simulink model "automata_learning"  (R2022a)
(part 8 of 10)

(exp(0.7734684944152832 * x2 - 0.6509665846824646 * x1 + 0.04056214913725853) - 1.0) / (exp(0.7734684944152832 * x2 - 0.6509665846824646 * x1 + 0.04056214913725853) + 1.0) + 0.0358128547668457 * (exp(0.018543146550655365 * x2 - 0.7226533889770508 * x1 + 0.3809460401535034) - 1.0) / (exp(0.018543146550655365 * x2 - 0.7226533889770508 * x1 + 0.3809460401535034) + 1.0) + 0.16037598252296448 * (exp(0.03828786686062813 * x1 + 0.43738114833831787 * x2 - 0.15343865752220154) - 1.0) / (exp(0.03828786686062813 * x1 + 0.43738114833831787 * x2 - 0.15343865752220154) + 1.0) + 0.879189133644104 * (exp(0.3266531825065613 * x1 + 0.7609410881996155 * x2 + 0.40537890791893005) - 1.0) / (exp(0.3266531825065613 * x1 + 0.7609410881996155 * x2 + 0.40537890791893005) + 1.0) + 0.47213396430015564 * (exp(0.20762847363948822 * x1 + 0.2858797609806061 * x2 - 0.43727564811706543) - 1.0) / (exp(0.20762847363948822 * x1 + 0.2858797609806061 * x2 - 0.43727564811706543) + 1.0) - 0.3890422284603119 * (exp(0.005666637327522039 * x1 + 0.6119794845581055 * x2 - 0.9893868565559387) - 1.0) / (exp(0.005666637327522039 * x1 + 0.6119794845581055 * x2 - 0.9893868565559387) + 1.0) + 0.4245724678039551 * (exp(0.39608341455459595 * x1 + 0.04428500309586525 * x2 + 0.2183447629213333) - 1.0) / (exp(0.39608341455459595 * x1 + 0.04428500309586525 * x2 + 0.2183447629213333) + 1.0) - 0.5148495435714722 * (exp(0.5634458065032959 * x1 - 0.8322378396987915 * x2 + 0.24965126812458038) - 1.0) / (exp(0.5634458065032959 * x1 - 0.8322378396987915 * x2 + 0.24965126812458038) + 1.0) - 0.5015235543251038 * (exp(0.3741709291934967 * x1 - 0.829635500907898 * x2 + 0.40845659375190735) - 1.0) / (exp(0.3741709291934967 * x1 - 0.829635500907898 * x2 + 0.40845659375190735) + 1.0) - 0.5266704559326172 * (exp(0.11800816655158997 * x2 - 0.6871803402900696 * x1 + 0.20091386139392853) - 1.0) / (exp(0.11800816655158997 * x2 - 0.6871803402900696 * x1 + 0.20091386139392853) + 1.0) - 0.6838598847389221 * (exp(0.19844788312911987 * x1 + 0.4046936631202698 * x2 - 0.9344500303268433) - 1.0) / (exp(0.19844788312911987 * x1 + 0.4046936631202698 * x2 - 0.9344500303268433) + 1.0) + 0.32724878191947937) + 1.0) - 0.29631882905960083 * (exp(0.33656391501426697 * (exp(0.5020318031311035 * x2 - 0.13788816332817078 * x1 + 0.02421402372419834) - 1.0) / (exp(0.5020318031311035 * x2 - 0.13788816332817078 * x1 + 0.02421402372419834) + 1.0) + 0.2108035683631897 * (exp(0.6166407465934753 * x1 + 1.262364149093628 * x2 + 0.2914634048938751) - 1.0) / (exp(0.6166407465934753 * x1 + 1.262364149093628 * x2 + 0.2914634048938751) + 1.0) + 0.5500431656837463 * (exp(0.03550431877374649 * x1 + 0.5916184186935425 * x2 - 0.08759552985429764) - 1.0) / (exp(0.03550431877374649 * x1 + 0.5916184186935425 * x2 - 0.08759552985429764) + 1.0) + 0.29068365693092346 * (exp(0.1657479703426361 * x1 - 0.679574728012085 * x2 + 0.5307417511940002) - 1.0) / (exp(0.1657479703426361 * x1 - 0.679574728012085 * x2 + 0.5307417511940002) + 1.0) + 0.6584247946739197 * (exp(0.14132575690746307 * x1 - 0.739913821220398 * x2 + 1.2046058177947998) - 1.0) / (exp(0.14132575690746307 * x1 - 0.739913821220398 * x2 + 1.2046058177947998) + 1.0) + 0.5027154088020325 * (exp(0.6150497794151306 * x1 - 0.6773995757102966 * x2 + 0.330721378326416) - 1.0) / (exp(0.6150497794151306 * x1 - 0.6773995757102966 * x2 + 0.330721378326416) + 1.0) - 0.6585365533828735 * (exp(0.3733357787132263 * x1 - 0.6249079704284668 * x2 + 0.3175375759601593) - 1.0) / (exp(0.3733357787132263 * x1 - 0.6249079704284668 * x2 + 0.3175375759601593) + 1.0) + 0.7110286951065063 * (exp(1.5124197006225586 * x1 + 1.2726414203643799 * x2 + 1.264981746673584) - 1.0) / (exp(1.5124197006225586 * x1 + 1.2726414203643799 * x2 + 1.264981746673584) + 1.0) + 0.14636917412281036 * (exp(0.6106719970703125 * x2 - 0.2651570439338684 * x1 + 0.22832649946212769) - 1.0) / (exp(0.6106719970703125 * x2 - 0.2651570439338684 * x1 + 0.22832649946212769) + 1.0) + 0.31852221488952637 * (exp(0.7734684944152832 * x2 - 0.6509665846824646 * x1 + 0.04056214913725853) - 1.0) / (exp(0.7734684944152832 * x2 - 0.6509665846824646 * x1 + 0.04056214913725853) + 1.0) + 0.049165740609169006 * (exp(0.018543146550655365 * x2 - 0.7226533889770508 * x1 + 0.3809460401535034) - 1.0) / (exp(0.018543146550655365 * x2 - 0.7226533889770508 * x1 + 0.3809460401535034) + 1.0) - 0.2836047410964966 * (exp(0.03828786686062813 * x1 + 0.43738114833831787 * x2 - 0.15343865752220154) - 1.0) / (exp(0.03828786686062813 * x1 + 0.43738114833831787 * x2 - 0.15343865752220154) + 1.0) - 0.5415816307067871 * (exp(0.3266531825065613 * x1 + 0.7609410881996155 * x2 + 0.40537890791893005) - 1.0) / (exp(0.3266531825065613 * x1 + 0.7609410881996155 * x2 + 0.40537890791893005) + 1.0) - 0.4399423599243164 * (exp(0.20762847363948822 * x1 + 0.2858797609806061 * x2 - 0.43727564811706543) - 1.0) / (exp(0.20762847363948822 * x1 + 0.2858797609806061 * x2 - 0.43727564811706543) + 1.0) - 0.0010141741950064898 * (exp(0.005666637327522039 * x1 + 0.6119794845581055 * x2 - 0.9893868565559387) - 1.0) / (exp(0.005666637327522039 * x1 + 0.6119794845581055 * x2 - 0.9893868565559387) + 1.0) + 0.5742956399917603 * (exp(0.39608341455459595 * x1 + 0.04428500309586525 * x2 + 0.2183447629213333) - 1.0) / (exp(0.39608341455459595 * x1 + 0.04428500309586525 * x2 + 0.2183447629213333) + 1.0) - 0.03165071830153465 * (exp(0.5634458065032959 * x1 - 0.8322378396987915 * x2 + 0.24965126812458038) - 1.0) / (exp(0.5634458065032959 * x1 - 0.8322378396987915 * x2 + 0.24965126812458038) + 1.0) - 0.6148557066917419 * (exp(0.3741709291934967 * x1 - 0.829635500907898 * x2 + 0.40845659375190735) - 1.0) / (exp(0.3741709291934967 * x1 - 0.829635500907898 * x2 + 0.40845659375190735) + 1.0) - 0.4349830448627472 * (exp(0.11800816655158997 * x2 - 0.6871803402900696 * x1 + 0.20091386139392853) - 1.0) / (exp(0.11800816655158997 * x2 - 0.6871803402900696 * x1 + 0.20091386139392853) + 1.0) + 0.4710049331188202 * (exp(0.19844788312911987 * x1 + 0.4046936631202698 * x2 - 0.9344500303268433) - 1.0) / (exp(0.19844788312911987 * x1 + 0.4046936631202698 * x2 - 0.9344500303268433) + 1.0) + 0.1878088265657425) - 1.0) / (exp(0.33656391501426697 * (exp(0.5020318031311035 * x2 - 0.13788816332817078 * x1 + 0.02421402372419834) - 1.0) / (exp(0.5020318031311035 * x2 - 0.13788816332817078 * x1 + 0.02421402372419834) + 1.0) + 0.2108035683631897 * (exp(0.6166407465934753 * x1 + 1.262364149093628 * x2 + 0.2914634048938751) - 1.0) / (exp(0.6166407465934753 * x1 + 1.262364149093628 * x2 + 0.2914634048938751) + 1.0) + 0.5500431656837463 * (exp(0.03550431877374649 * x1 + 0.5916184186935425 * x2 - 0.08759552985429764) - 1.0) / (exp(0.03550431877374649 * x1 + 0.5916184186935425 * x2 - 0.08759552985429764) + 1.0) + 0.29068365693092346 * (exp(0.1657479703426361 * x1 - 0.679574728012085 * x2 + 0.5307417511940002) - 1.0) / (exp(0.1657479703426361 * x1 - 0.679574728012085 * x2 + 0.5307417511940002) + 1.0) + 0.6584247946739197 * (exp(0.14132575690746307 * x1 - 0.739913821220398 * x2 + 1.2046058177947998) - 1.0) / (exp(0.14132575690746307 * x1 - 0.739913821220398 * x2 + 1.2046058177947998) + 1.0) + 0.5027154088020325 * (exp(0.6150497794151306 * x1 - 0.6773995757102966 * x2 + 0.330721378326416) - 1.0) / (exp(0.6150497794151306 * x1 - 0.6773995757102966 * x2 + 0.330721378326416) + 1.0) - 0.6585365533828735 * (exp(0.3733357787132263 * x1 - 0.6249079704284668 * x2 + 0.3175375759601593) - 1.0) / (exp(0.3733357787132263 * x1 - 0.6249079704284668 * x2 + 0.3175375759601593) + 1.0) + 0.7110286951065063 * (exp(1.5124197006225586 * x1 + 1.2726414203643799 * x2 + 1.264981746673584) - 1.0) / (exp(1.5124197006225586 * x1 + 1.2726414203643799 * x2 + 1.264981746673584) + 1.0) + 0.14636917412281036 * (exp(0.6106719970703125 * x2 - 0.2651570439338684 * x1 + 0.22832649946212769) - 1.0) / (exp(0.6106719970703125 * x2 - 0.2651570439338684 * x1 + 0.22832649946212769) + 1.0) + 0.31852221488952637 * (exp(0.7734684944152832 * x2 - 0.6509665846824646 * x1 + 0.04056214913725853) - 1.0) / (exp(0.7734684944152832 * x2 - 0.6509665846824646 * x1 + 0.04056214913725853) + 1.0) + 0.049165740609169006 * (exp(0.018543146550655365 * x2 - 0.7226533889770508 * x1 + 0.3809460401535034) - 1.0) / (exp(0.018543146550655365 * x2 - 0.7226533889770508 * x1 + 0.3809460401535034) + 1.0) - 0.2836047410964966 * (exp(0.03828786686062813 * x1 + 0.43738114833831787 * x2 - 0.15343865752220154) - 1.0) / (exp(0.03828786686062813 * x1 + 0.43738114833831787 * x2 - 0.15343865752220154) + 1.0) - 0.5415816307067871 * (exp(0.3266531825065613 * x1 + 0.7609410881996155 * x2 + 0.40537890791893005) - 1.0) / (exp(0.3266531825065613 * x1 + 0.7609410881996155 * x2 + 0.40537890791893005) + 1.0) - 0.4399423599243164 * (exp(0.20762847363948822 * x1 + 0.2858797609806061 * x2 - 0.43727564811706543) - 1.0) / (exp(0.20762847363948822 * x1 + 0.2858797609806061 * x2 - 0.43727564811706543) + 1.0) - 0.0010141741950064898 * (exp(0.005666637327522039 * x1 + 0.6119794845581055 * x2 - 0.9893868565559387) - 1.0) / (exp(0.005666637327522039 * x1 + 0.6119794845581055 * x2 - 0.9893868565559387) + 1.0) + 0.5742956399917603 * (exp(0.39608341455459595 * x1 + 0.04428500309586525 * x2 + 0.2183447629213333) - 1.0) / (exp(0.39608341455459595 * x1 + 0.04428500309586525 * x2 + 0.2183447629213333) + 1.0) - 0.03165071830153465 * (exp(0.5634458065032959 * x1 - 0.8322378396987915 * x2 + 0.24965126812458038) - 1.0) / (exp(0.5634458065032959 * x1 - 0.8322378396987915 * x2 + 0.24965126812458038) + 1.0) - 0.6148557066917419 * (exp(0.3741709291934967 * x1 - 0.829635500907898 * x2 + 0.40845659375190735) - 1.0) / (exp(0.3741709291934967 * x1 - 0.829635500907898 * x2 + 0.40845659375190735) + 1.0) - 0.4349830448627472 * (exp(0.11800816655158997 * x2 - 0.6871803402900696 * x1 + 0.20091386139392853) - 1.0) / (exp(0.11800816655158997 * x2 - 0.6871803402900696 * x1 + 0.20091386139392853) + 1.0) + 0.4710049331188202 * (exp(0.19844788312911987 * x1 + 0.4046936631202698 * x2 - 0.9344500303268433) - 1.0) / (exp(0.19844788312911987 * x1 + 0.4046936631202698 * x2 - 0.9344500303268433) + 1.0) + 0.1878088265657425) + 1.0) - 0.2150561660528183 * (exp(0.02026395872235298 * (exp(0.6166407465934753 * x1 + 1.262364149093628 * x2 + 0.2914634048938751) - 1.0) / (exp(0.6166407465934753 * x1 + 1.262364149093628 * x2 + 0.2914634048938751) + 1.0) - 0.03688286617398262 * (exp(0.5020318031311035 * x2 - 0.13788816332817078 * x1 + 0.02421402372419834) - 1.0) / (exp(0.5020318031311035 * x2 - 0.13788816332817078 * x1 + 0.02421402372419834) + 1.0) + 0.8227269649505615 * (exp(0.03550431877374649 * x1 + 0.5916184186935425 * x2 - 0.08759552985429764) - 1.0) / (exp(0.03550431877374649 * x1 + 0.5916184186935425 * x2 - 0.08759552985429764) + 1.0) + 0.10660602152347565 * (exp(0.1657479703426361 * x1 - 0.679574728012085 * x2 + 0.5307417511940002) - 1.0) / (exp(0.1657479703426361 * x1 - 0.679574728012085 * x2 + 0.5307417511940002) + 1.0) + 0.0043801916763186455 * (exp(0.14132575690746307 * x1 - 0.739913821220398 * x2 + 1.2046058177947998) - 1.0) / (exp(0.14132575690746307 * x1 - 0.739913821220398 * x2 + 1.2046058177947998) + 1.0) + 0.174507275223732 * (exp(0.6150497794151306 * x1 - 0.6773995757102966 * x2 + 0.330721378326416) - 1.0) / (exp(0.6150497794151306 * x1 - 0.6773995757102966 * x2 + 0.330721378326416) + 1.0) + 0.2544170916080475 * (exp(0.3733357787132263 * x1 - 0.6249079704284668 * x2 + 0.3175375759601593) - 1.0) / (exp(0.3733357787132263 * x1 - 0.6249079704284668 * x2 + 0.3175375759601593) + 1.0) + 0.7126232385635376 * (exp(1.5124197006225586 * x1 + 1.2726414203643799 * x2 + 1.264981746673584) - 1.0) / (exp(1.5124197006225586 * x1 + 1.2726414203643799 * x2 + 1.264981746673584) + 1.0) + 0.23010414838790894 * (exp(0.6106719970703125 * x2 - 0.2651570439338684 * x1 + 0.22832649946212769) - 1.0) / (exp(0.6106719970703125 * x2 - 0.2651570439338684 * x1 + 0.22832649946212769) + 1.0) + 0.5714036226272583 * (exp(0.7734684944152832 * x2 - 0.6509665846824646 * x1 + 0.04056214913725853) - 1.0) / (exp(0.7734684944152832 * x2 - 0.6509665846824646 * x1 + 0.04056214913725853) + 1.0) + 0.5201306939125061 * (exp(0.018543146550655365 * x2 - 0.7226533889770508 * x1 + 0.3809460401535034) - 1.0) / (exp(0.018543146550655365 * x2 - 0.7226533889770508 * x1 + 0.3809460401535034) + 1.0) + 0.23737752437591553 * (exp(0.03828786686062813 * x1 + 0.43738114833831787 * x2 - 0.15343865752220154) - 1.0) / (exp(0.03828786686062813 * x1 + 0.43738114833831787 * x2 - 0.15343865752220154) + 1.0) + 0.3255254924297333 * (exp(0.3266531825065613 * x1 + 0.7609410881996155 * x2 + 0.40537890791893005) - 1.0) / (exp(0.3266531825065613 * x1 + 0.7609410881996155 * x2 + 0.40537890791893005) + 1.0) - 0.5285819172859192 * (exp(0.20762847363948822 * x1 + 0.2858797609806061 * x2 - 0.43727564811706543) - 1.0) / (exp(0.20762847363948822 * x1 + 0.2858797609806061 * x2 - 0.43727564811706543) + 1.0) + 0.8047150373458862 * (exp(0.005666637327522039 * x1 + 0.6119794845581055 * x2 - 0.9893868565559387) - 1.0) / (exp(0.005666637327522039 * x1 + 0.6119794845581055 * x2 - 0.9893868565559387) + 1.0) + 0.17543937265872955 * (exp(0.39608341455459595 * x1 + 0.04428500309586525 * x2 + 0.2183447629213333) - 1.0) / (exp(0.39608341455459595 * x1 + 0.04428500309586525 * x2 + 0.2183447629213333) + 1.0) - 0.8977094888687134 * (exp(0.5634458065032959 * x1 - 0.8322378396987915 * x2 + 0.24965126812458038) - 1.0) / (exp(0.5634458065032959 * x1 - 0.8322378396987915 * x2 + 0.24965126812458038) + 1.0) + 0.4383457601070404 * (exp(0.3741709291934967 * x1 - 0.829635500907898 * x2 + 0.40845659375190735) - 1.0) / (exp(0.3741709291934967 * x1 - 0.829635500907898 * x2 + 0.40845659375190735) + 1.0) + 0.23758132755756378 * (exp(0.11800816655158997 * x2 - 0.6871803402900696 * x1 + 0.20091386139392853) - 1.0) / (exp(0.11800816655158997 * x2 - 0.6871803402900696 * x1 + 0.20091386139392853) + 1.0) - 0.07985717803239822 * (exp(0.19844788312911987 * x1 + 0.4046936631202698 * x2 - 0.9344500303268433) - 1.0) / (exp(0.19844788312911987 * x1 + 0.4046936631202698 * x2 - 0.9344500303268433) + 1.0) + 0.2756956219673157) - 1.0) / (exp(0.02026395872235298 * (exp(0.6166407465934753 * x1 + 1.262364149093628 * x2 + 0.2914634048938751) - 1.0) / (exp(0.6166407465934753 * x1 + 1.262364149093628 * x2 + 0.2914634048938751) + 1.0) - 0.03688286617398262 * (exp(0.5020318031311035 * x2 - 0.13788816332817078 * x1 + 0.02421402372419834) - 1.0) / (exp(0.5020318031311035 * x2 - 0.13788816332817078 * x1 + 0.02421402372419834) + 1.0) + 0.8227269649505615 * (exp(0.03550431877374649 * x1 + 0.5916184186935425 * x2 - 0.08759552985429764) - 1.0) / (exp(0.03550431877374649 * x1 + 0.5916184186935425 * x2 - 0.08759552985429764) + 1.0) + 0.10660602152347565 * (exp(0.1657479703426361 * x1 - 0.679574728012085 * x2 + 0.5307417511940002) - 1.0) / (exp(0.1657479703426361 * x1 - 0.679574728012085 * x2 + 0.5307417511940002) + 1.0) + 0.0043801916763186455 * (exp(0.14132575690746307 * x1 - 0.739913821220398 * x2 + 1.2046058177947998) - 1.0) / (exp(0.14132575690746307 * x1 - 0.739913821220398 * x2 + 1.2046058177947998) + 1.0) + 0.174507275223732 * (exp(0.6150497794151306 * x1 - 0.6773995757102966 * x2 + 0.330721378326416) - 1.0) / (exp(0.6150497794151306 * x1 - 0.6773995757102966 * x2 + 0.330721378326416) + 1.0) + 0.2544170916080475 * (exp(0.3733357787132263 * x1 - 0.6249079704284668 * x2 + 0.3175375759601593) - 1.0) / (exp(0.3733357787132263 * x1 - 0.6249079704284668 * x2 + 0.3175375759601593) + 1.0) + 0.7126232385635376 * (exp(1.5124197006225586 * x1 + 1.2726414203643799 * x2 + 1.264981746673584) - 1.0) / (exp(1.5124197006225586 * x1 + 1.2726414203643799 * x2 + 1.264981746673584) + 1.0) + 0.23010414838790894 * (exp(0.6106719970703125 * x2 - 0.2651570439338684 * x1 + 0.22832649946212769) - 1.0) / (exp(0.6106719970703125 * x2 - 0.2651570439338684 * x1 + 0.22832649946212769) + 1.0) + 0.5714036226272583 * (exp(0.7734684944152832 * x2 - 0.6509665846824646 * x1 + 0.04056214913725853) - 1.0) / (exp(0.7734684944152832 * x2 - 0.6509665846824646 * x1 + 0.04056214913725853) + 1.0) + 0.5201306939125061 * (exp(0.018543146550655365 * x2 - 0.7226533889770508 * x1 + 0.3809460401535034) - 1.0) / (exp(0.018543146550655365 * x2 - 0.7226533889770508 * x1 + 0.3809460401535034) + 1.0) + 0.23737752437591553 * (exp(0.03828786686062813 * x1 + 0.43738114833831787 * x2 - 0.15343865752220154) - 1.0) / (exp(0.03828786686062813 * x1 + 0.43738114833831787 * x2 - 0.15343865752220154) + 1.0) + 0.3255254924297333 * (exp(0.3266531825065613 * x1 + 0.7609410881996155 * x2 + 0.40537890791893005) - 1.0) / (exp(0.3266531825065613 * x1 + 0.7609410881996155 * x2 + 0.40537890791893005) + 1.0) - 0.5285819172859192 * (exp(0.20762847363948822 * x1 + 0.2858797609806061 * x2 - 0.43727564811706543) - 1.0) / (exp(0.20762847363948822 * x1 + 0.2858797609806061 * x2 - 0.43727564811706543) + 1.0) + 0.8047150373458862 * (exp(0.005666637327522039 * x1 + 0.6119794845581055 * x2 - 0.9893868565559387) - 1.0) / (exp(0.005666637327522039 * x1 + 0.6119794845581055 * x2 - 0.9893868565559387) + 1.0) + 0.17543937265872955 * (exp(0.39608341455459595 * x1 + 0.04428500309586525 * x2 + 0.2183447629213333) - 1.0) / (exp(0.39608341455459595 * x1 + 0.04428500309586525 * x2 + 0.2183447629213333) + 1.0) - 0.8977094888687134 * (exp(0.5634458065032959 * x1 - 0.8322378396987915 * x2 + 0.24965126812458038) - 1.0) / (exp(0.5634458065032959 * x1 - 0.8322378396987915 * x2 + 0.24965126812458038) + 1.0) + 0.4383457601070404 * (exp(0.3741709291934967 * x1 - 0.829635500907898 * x2 + 0.40845659375190735) - 1.0) / (exp(0.3741709291934967 * x1 - 0.829635500907898 * x2 + 0.40845659375190735) + 1.0) + 0.23758132755756378 * (exp(0.11800816655158997 * x2 - 0.6871803402900696 * x1 + 0.20091386139392853) - 1.0) / (exp(0.11800816655158997 * x2 - 0.6871803402900696 * x1 + 0.20091386139392853) + 1.0) - 0.07985717803239822 * (exp(0.19844788312911987 * x1 + 0.4046936631202698 * x2 - 0.9344500303268433) - 1.0) / (exp(0.19844788312911987 * x1 + 0.4046936631202698 * x2 - 0.9344500303268433) + 1.0) + 0.2756956219673157) + 1.0) - 0.1457960605621338;
